simulink library "SimulinkForSyDe"  (R2020b)
settings: Solver=VariableStepAuto  StartTime=0.0  StopTime=10.0  RelTol=1e-3
undefined symbols (not defined in the file): __PRM__SERIALIZED__DATA__, delaynSY
settings Model: Creator=Andrea  LastModifiedBy=Andrea

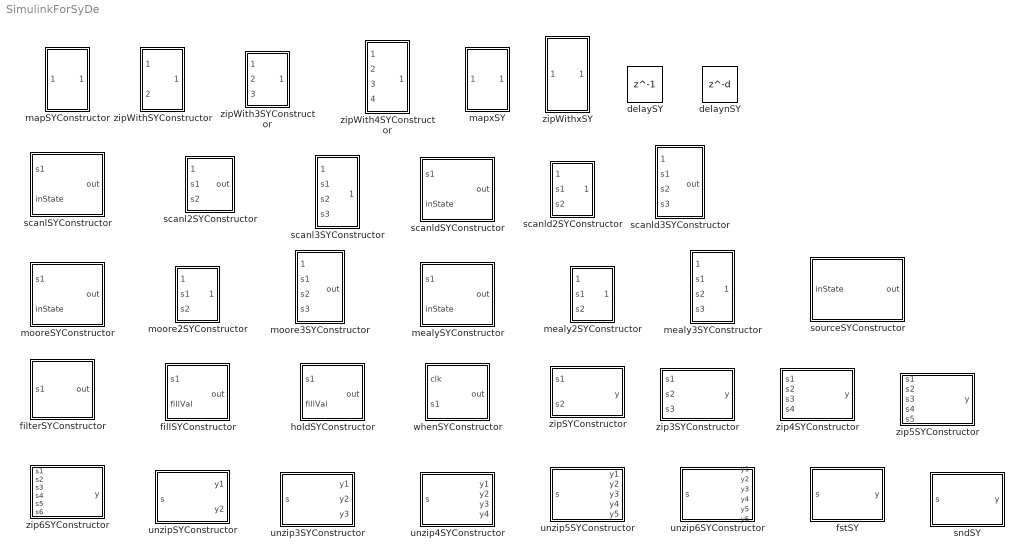
== system SimulinkForSyDe ==
  delaySY : Delay  BlockKeywords=__PRM__SERIALIZED__DATA__:My Integrator  DelayLength=1  InitialConditionSource=Input port
      settings: InputPortMap=u0,p4
  delaynSY : Delay  BlockKeywords=__PRM__SERIALIZED__DATA__:delaynSY  DelayLengthSource=Input port  DelayLength=1  InitialConditionSource=Input port
      settings: InputPortMap=u0,p1,p4
  fillSYConstructor : Stateflow chart  Description="Signals with NaN values cannot be easily imported from Matlab to Simulink and this block need clean signal as input (you  can use cleanNanScript to clean the input signal)."  TreatAsAtomicUnit=on
  filterSYConstructor : Subsystem  Description=The limit must be decided inside the Simulink's function block. The template is equivalent to: filterSY (<=3) s1
  fstSY : MATLAB Function  TreatAsAtomicUnit=on
  holdSYConstructor : Stateflow chart  TreatAsAtomicUnit=on
  mapSYConstructor : Subsystem
  mapxSY : Subsystem  Description=the input must be a mux of signals and the sum is the function used as example
  mealy2SYConstructor : Subsystem
  mealy3SYConstructor : Subsystem
  mealySYConstructor : Subsystem  Description=|
      | The combinational function for next state decoder and for the output have to be set inside this subsystem (disabing the links).
      | This block is a template corresponding to the ForSyDe line of code: mealySY (+) (*) inState $ s1
  moore2SYConstructor : Subsystem
  moore3SYConstructor : Subsystem
  mooreSYConstructor : Subsystem  Description=|
      | The combinational function for next state decoder and for the output have to be set inside this subsystem (disabing the links).
      | This block is a template corresponding to the ForSyDe line of code: mooreSY (+) (*2) inState $ s1.
  scanl2SYConstructor : Subsystem
  scanl3SYConstructor : Subsystem
  scanlSYConstructor : Subsystem  Description=|
      | The combinational function for the output have to be set inside this subsystem (disabing the links).
      | This block is a template corresponding to the ForSyDe line of code: scanlSY (+) inState s1
  scanld2SYConstructor : Subsystem
  scanld3SYConstructor : Subsystem
  scanldSYConstructor : Subsystem  Description=|
      | The combinational function for next state decoder has to be set inside this subsystem (disabing the links).
      | This block is a template corresponding to the ForSyDe line of code: scanldSY (+) inState s1
  sndSY : MATLAB Function  TreatAsAtomicUnit=on
  sourceSYConstructor : Subsystem  Description=The recurrent function has to be changed inside the SImulink's function block. The default template is equivalent to: sourceSY (+1) 0
  unzip3SYConstructor : MATLAB Function  TreatAsAtomicUnit=on
  unzip4SYConstructor : MATLAB Function  TreatAsAtomicUnit=on
  unzip5SYConstructor : MATLAB Function  TreatAsAtomicUnit=on
  unzip6SYConstructor : MATLAB Function  TreatAsAtomicUnit=on
  unzipSYConstructor : MATLAB Function  TreatAsAtomicUnit=on
  whenSYConstructor : Stateflow chart  TreatAsAtomicUnit=on
  zip3SYConstructor : MATLAB Function  TreatAsAtomicUnit=on
  zip4SYConstructor : MATLAB Function  TreatAsAtomicUnit=on
  zip5SYConstructor : MATLAB Function  TreatAsAtomicUnit=on
  zip6SYConstructor : MATLAB Function  TreatAsAtomicUnit=on
  zipSYConstructor : MATLAB Function  TreatAsAtomicUnit=on
  zipWith3SYConstructor : Subsystem
  zipWith4SYConstructor : Subsystem
  zipWithSYConstructor : Subsystem
  zipWithxSY : Subsystem  Description=xSig must be defined before using this block from Matlab and indicates the number of signals contained in the input signals vector

== system SimulinkForSyDe/filterSYConstructor ==
  s1 : Inport
  filterSY : Stateflow chart  TreatAsAtomicUnit=on
  filterf : Subsystem  TreatAsAtomicUnit=on
  out : Outport
  wires:
  filterSY/1(out) -> out/1
  s1/1 -> filterSY/1(s1)

== system SimulinkForSyDe/mapSYConstructor ==
  In1 : Inport
  mapSY : FunctionCaller  FunctionPrototype=y = mapSYf(u)  InputArgumentSpecifications=<Enter example>  OutputArgumentSpecifications=<Enter example>
  mapSY Function : Subsystem  TreatAsAtomicUnit=on
  Out1 : Outport
  wires:
  In1/1 -> mapSY/1
  mapSY/1 -> Out1/1

== system SimulinkForSyDe/mapxSY ==
  In1 : Inport
  Constant : Constant
  Sum : Sum  Inputs=|++
  Out1 : Outport
  wires:
  In1/1 -> Sum/1
  Sum/1 -> Out1/1
  Constant/1 -> Sum/2

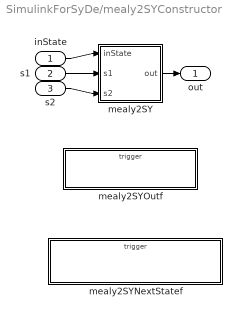
== system SimulinkForSyDe/mealy2SYConstructor ==
  inState : Inport
  s1 : Inport  Port=2
  s2 : Inport  Port=3
  mealy2SY : Stateflow chart  TreatAsAtomicUnit=on
  mealy2SYNextStatef : Subsystem  TreatAsAtomicUnit=on
  mealy2SYOutf : Subsystem  TreatAsAtomicUnit=on
  out : Outport
  wires:
  inState/1 -> mealy2SY/1(inState)
  s1/1 -> mealy2SY/2(s1)
  s2/1 -> mealy2SY/3(s2)
  mealy2SY/1(out) -> out/1

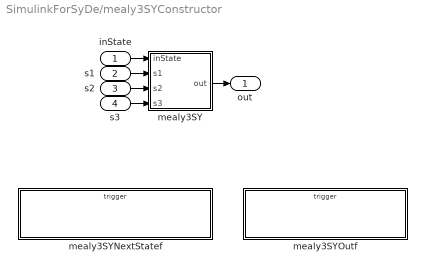
== system SimulinkForSyDe/mealy3SYConstructor ==
  inState : Inport
  s1 : Inport  Port=2
  s2 : Inport  Port=3
  s3 : Inport  Port=4
  mealy3SY : Stateflow chart  TreatAsAtomicUnit=on
  mealy3SYNextStatef : Subsystem  TreatAsAtomicUnit=on
  mealy3SYOutf : Subsystem  TreatAsAtomicUnit=on
  out : Outport
  wires:
  s3/1 -> mealy3SY/4(s3)
  s1/1 -> mealy3SY/2(s1)
  mealy3SY/1(out) -> out/1
  s2/1 -> mealy3SY/3(s2)
  inState/1 -> mealy3SY/1(inState)

== system SimulinkForSyDe/mealySYConstructor ==
  s1 : Inport
  inState : Inport  Port=2
  mealySY : Stateflow chart  TreatAsAtomicUnit=on
  mealySYNextStatef : Subsystem  TreatAsAtomicUnit=on
  mealySYOutf : Subsystem  TreatAsAtomicUnit=on
  out : Outport
  wires:
  mealySY/1(out) -> out/1
  s1/1 -> mealySY/1(s1)
  inState/1 -> mealySY/2(inState)

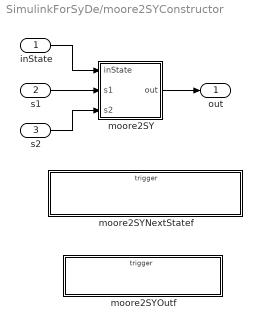
== system SimulinkForSyDe/moore2SYConstructor ==
  inState : Inport
  s1 : Inport  Port=2
  s2 : Inport  Port=3
  moore2SY : Stateflow chart  TreatAsAtomicUnit=on
  moore2SYNextStatef : Subsystem  TreatAsAtomicUnit=on
  moore2SYOutf : Subsystem  TreatAsAtomicUnit=on
  out : Outport
  wires:
  inState/1 -> moore2SY/1(inState)
  s2/1 -> moore2SY/3(s2)
  moore2SY/1(out) -> out/1
  s1/1 -> moore2SY/2(s1)

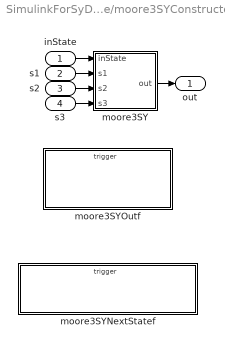
== system SimulinkForSyDe/moore3SYConstructor ==
  inState : Inport
  s1 : Inport  Port=2
  s2 : Inport  Port=3
  s3 : Inport  Port=4
  moore3SY : Stateflow chart  TreatAsAtomicUnit=on
  moore3SYNextStatef : Subsystem  TreatAsAtomicUnit=on
  moore3SYOutf : Subsystem  TreatAsAtomicUnit=on
  out : Outport
  wires:
  moore3SY/1(out) -> out/1
  s1/1 -> moore3SY/2(s1)
  inState/1 -> moore3SY/1(inState)
  s2/1 -> moore3SY/3(s2)
  s3/1 -> moore3SY/4(s3)

== system SimulinkForSyDe/mooreSYConstructor ==
  s1 : Inport
  inState : Inport  Port=2
  mooreSY : Stateflow chart  TreatAsAtomicUnit=on
  mooreSYNextStatef : Subsystem  TreatAsAtomicUnit=on
  mooreSYOutf : Subsystem  TreatAsAtomicUnit=on
  out : Outport
  wires:
  s1/1 -> mooreSY/1(s1)
  inState/1 -> mooreSY/2(inState)
  mooreSY/1(out) -> out/1

== system SimulinkForSyDe/scanl2SYConstructor ==
  inState : Inport
  s1 : Inport  Port=2
  s2 : Inport  Port=3
  scanl2SY : Stateflow chart  TreatAsAtomicUnit=on
  scanl2SYOutf : Subsystem  TreatAsAtomicUnit=on
  out : Outport
  wires:
  s2/1 -> scanl2SY/3(s2)
  inState/1 -> scanl2SY/1(inState)
  s1/1 -> scanl2SY/2(s1)
  scanl2SY/1(out) -> out/1

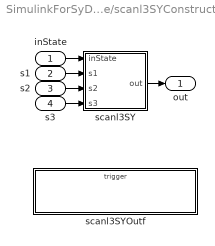
== system SimulinkForSyDe/scanl3SYConstructor ==
  inState : Inport
  s1 : Inport  Port=2
  s2 : Inport  Port=3
  s3 : Inport  Port=4
  scanl3SY : Stateflow chart  TreatAsAtomicUnit=on
  scanl3SYOutf : Subsystem  TreatAsAtomicUnit=on
  out : Outport
  wires:
  s2/1 -> scanl3SY/3(s2)
  s1/1 -> scanl3SY/2(s1)
  inState/1 -> scanl3SY/1(inState)
  scanl3SY/1(out) -> out/1
  s3/1 -> scanl3SY/4(s3)

== system SimulinkForSyDe/scanlSYConstructor ==
  s1 : Inport
  inState : Inport  Port=2
  scanlSY : Stateflow chart  TreatAsAtomicUnit=on
  scanlSYOutf : Subsystem  TreatAsAtomicUnit=on
  out : Outport
  wires:
  scanlSY/1(out) -> out/1
  s1/1 -> scanlSY/1(s1)
  inState/1 -> scanlSY/2(inState)

== system SimulinkForSyDe/scanld2SYConstructor ==
  inState : Inport
  s1 : Inport  Port=2
  s2 : Inport  Port=3
  scanld2SY : Stateflow chart  TreatAsAtomicUnit=on
  scanld2SYNextf : Subsystem  TreatAsAtomicUnit=on
  out : Outport
  wires:
  s1/1 -> scanld2SY/2(s1)
  inState/1 -> scanld2SY/1(inState)
  scanld2SY/1(out) -> out/1
  s2/1 -> scanld2SY/3(s2)

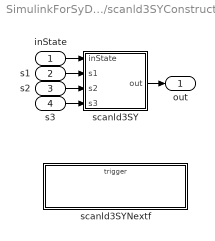
== system SimulinkForSyDe/scanld3SYConstructor ==
  inState : Inport
  s1 : Inport  Port=2
  s2 : Inport  Port=3
  s3 : Inport  Port=4
  scanld3SY : Stateflow chart  TreatAsAtomicUnit=on
  scanld3SYNextf : Subsystem  TreatAsAtomicUnit=on
  out : Outport
  wires:
  s3/1 -> scanld3SY/4(s3)
  s1/1 -> scanld3SY/2(s1)
  s2/1 -> scanld3SY/3(s2)
  scanld3SY/1(out) -> out/1
  inState/1 -> scanld3SY/1(inState)

== system SimulinkForSyDe/scanldSYConstructor ==
  s1 : Inport
  inState : Inport  Port=2
  scanldSY : Stateflow chart  Description=|  TreatAsAtomicUnit=on
      | The combinational function for next state decoder cannot be given as input and the block itself has to be modified to set the wanted decoder function. 
      | This block is a template corresponding to the ForSyDe line of code: scanldSY (+) inState s1
  scanldSYNextf : Subsystem  TreatAsAtomicUnit=on
  out : Outport
  wires:
  s1/1 -> scanldSY/1(s1)
  inState/1 -> scanldSY/2(inState)
  scanldSY/1(out) -> out/1

== system SimulinkForSyDe/sourceSYConstructor ==
  inState : Inport
  To Workspace1 : ToWorkspace  VariableName=yOut  SampleTime=-1
      settings: Save2DSignal=2-D array (concatenate along first dimension)
  recursivef : Subsystem  TreatAsAtomicUnit=on
  sourceSY : Stateflow chart  TreatAsAtomicUnit=on
  out : Outport
  wires:
  inState/1 -> sourceSY/1(inState)
  sourceSY/1(out) -> To Workspace1/1, out/1

== system SimulinkForSyDe/zipWith3SYConstructor ==
  In1 : Inport
  In2 : Inport  Port=2
  In3 : Inport  Port=3
  zipWith3SY : FunctionCaller  FunctionPrototype=y = zipWith3SYf(u,u1,u2)  InputArgumentSpecifications=<Enter example>  OutputArgumentSpecifications=<Enter example>
  zipWith3SY caller : Subsystem  TreatAsAtomicUnit=on
  Out1 : Outport
  wires:
  zipWith3SY/1 -> Out1/1
  In1/1 -> zipWith3SY/1
  In3/1 -> zipWith3SY/3
  In2/1 -> zipWith3SY/2

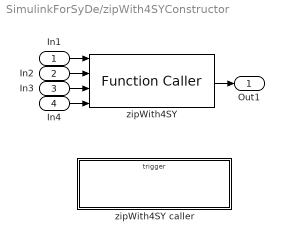
== system SimulinkForSyDe/zipWith4SYConstructor ==
  In1 : Inport
  In2 : Inport  Port=2
  In3 : Inport  Port=3
  In4 : Inport  Port=4
  zipWith4SY : FunctionCaller  FunctionPrototype=y = zipWith4SYf(u,u1,u2,u3)  InputArgumentSpecifications=<Enter example>  OutputArgumentSpecifications=<Enter example>
  zipWith4SY caller : Subsystem  TreatAsAtomicUnit=on
  Out1 : Outport
  wires:
  In2/1 -> zipWith4SY/2
  In1/1 -> zipWith4SY/1
  zipWith4SY/1 -> Out1/1
  In3/1 -> zipWith4SY/3
  In4/1 -> zipWith4SY/4

== system SimulinkForSyDe/zipWithSYConstructor ==
  In1 : Inport
  In2 : Inport  Port=2
  zipWithSY : FunctionCaller  FunctionPrototype=y = zipWithSYf(u,u1)  InputArgumentSpecifications=<Enter example>  OutputArgumentSpecifications=<Enter example>
  zipWithSY caller : Subsystem  TreatAsAtomicUnit=on
  Out1 : Outport
  wires:
  In1/1 -> zipWithSY/1
  zipWithSY/1 -> Out1/1
  In2/1 -> zipWithSY/2

== system SimulinkForSyDe/zipWithxSY ==
  In1 : Inport
  Demux : Demux  Outputs=3
  Sum : Sum  Inputs=+++
  Out3 : Outport
  wires:
  Demux/1 -> Sum/1
  Sum/1 -> Out3/1
  Demux/2 -> Sum/2
  Demux/3 -> Sum/3
  In1/1 -> Demux/1

== system SimulinkForSyDe/filterSYConstructor/filterf ==
  filterf : TriggerPort  TriggerType=function-call  IsSimulinkFunction=on  FunctionName=filterf  FunctionVisibility=scoped  VariantControl=(inherit)
  Constant1 : Constant  Value=3
  Sum : Sum  Inputs=|+-
  u : ArgIn  DisableCoverage=on  ArgumentName=u
  y : ArgOut  DisableCoverage=on  ArgumentName=y
  wires:
  u/1 -> Sum/1
  Constant1/1 -> Sum/2
  Sum/1 -> y/1

== system SimulinkForSyDe/mapSYConstructor/mapSY Function ==
  mapSYf : TriggerPort  TriggerType=function-call  IsSimulinkFunction=on  FunctionName=mapSYf  FunctionVisibility=scoped  VariantControl=(inherit)
  Constant : Constant
  Sum : Sum  Inputs=|++
  u : ArgIn  DisableCoverage=on  ArgumentName=u
  y : ArgOut  DisableCoverage=on  ArgumentName=y
  wires:
  Constant/1 -> Sum/2
  u/1 -> Sum/1
  Sum/1 -> y/1

== system SimulinkForSyDe/mealy2SYConstructor/mealy2SYNextStatef ==
  mealy2SYNextStatef : TriggerPort  TriggerType=function-call  IsSimulinkFunction=on  FunctionName=mealy2SYNextStatef  FunctionVisibility=scoped  VariantControl=(inherit)
  Sum : Sum  Inputs=+++
  u : ArgIn  DisableCoverage=on  ArgumentName=u
  u1 : ArgIn  DisableCoverage=on  Port=2  ArgumentName=u1
  u2 : ArgIn  DisableCoverage=on  Port=3  ArgumentName=u2
  y : ArgOut  DisableCoverage=on  ArgumentName=y
  wires:
  u1/1 -> Sum/2
  Sum/1 -> y/1
  u/1 -> Sum/1
  u2/1 -> Sum/3

== system SimulinkForSyDe/mealy2SYConstructor/mealy2SYOutf ==
  mealy2SYOutf : TriggerPort  TriggerType=function-call  IsSimulinkFunction=on  FunctionName=mealy2SYOutf  FunctionVisibility=scoped  VariantControl=(inherit)
  Sum : Sum  Inputs=+++
  u : ArgIn  DisableCoverage=on  ArgumentName=u
  u1 : ArgIn  DisableCoverage=on  Port=2  ArgumentName=u1
  u2 : ArgIn  DisableCoverage=on  Port=3  ArgumentName=u2
  y : ArgOut  DisableCoverage=on  ArgumentName=y
  wires:
  u1/1 -> Sum/2
  Sum/1 -> y/1
  u/1 -> Sum/1
  u2/1 -> Sum/3

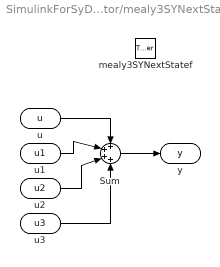
== system SimulinkForSyDe/mealy3SYConstructor/mealy3SYNextStatef ==
  mealy3SYNextStatef : TriggerPort  TriggerType=function-call  IsSimulinkFunction=on  FunctionName=mealy3SYNextStatef  FunctionVisibility=scoped  VariantControl=(inherit)
  Sum : Sum  Inputs=++++
  u : ArgIn  DisableCoverage=on  ArgumentName=u
  u1 : ArgIn  DisableCoverage=on  Port=2  ArgumentName=u1
  u2 : ArgIn  DisableCoverage=on  Port=3  ArgumentName=u2
  u3 : ArgIn  DisableCoverage=on  Port=4  ArgumentName=u3
  y : ArgOut  DisableCoverage=on  ArgumentName=y
  wires:
  u1/1 -> Sum/2
  u/1 -> Sum/1
  u2/1 -> Sum/3
  Sum/1 -> y/1
  u3/1 -> Sum/4

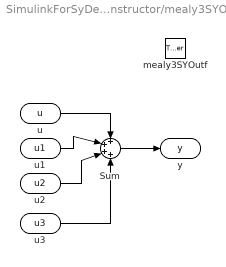
== system SimulinkForSyDe/mealy3SYConstructor/mealy3SYOutf ==
  mealy3SYOutf : TriggerPort  TriggerType=function-call  IsSimulinkFunction=on  FunctionName=mealy3SYOutf  FunctionVisibility=scoped  VariantControl=(inherit)
  Sum : Sum  Inputs=++++
  u : ArgIn  DisableCoverage=on  ArgumentName=u
  u1 : ArgIn  DisableCoverage=on  Port=2  ArgumentName=u1
  u2 : ArgIn  DisableCoverage=on  Port=3  ArgumentName=u2
  u3 : ArgIn  DisableCoverage=on  Port=4  ArgumentName=u3
  y : ArgOut  DisableCoverage=on  ArgumentName=y
  wires:
  u1/1 -> Sum/2
  u/1 -> Sum/1
  u2/1 -> Sum/3
  Sum/1 -> y/1
  u3/1 -> Sum/4

== system SimulinkForSyDe/mealySYConstructor/mealySYNextStatef ==
  mealySYNextStatef : TriggerPort  TriggerType=function-call  IsSimulinkFunction=on  FunctionName=mealySYNextStatef  FunctionVisibility=scoped  VariantControl=(inherit)
  Sum : Sum  Inputs=|++
  u : ArgIn  DisableCoverage=on  ArgumentName=u
  u1 : ArgIn  DisableCoverage=on  Port=2  ArgumentName=u1
  y : ArgOut  DisableCoverage=on  ArgumentName=y
  wires:
  u/1 -> Sum/1
  u1/1 -> Sum/2
  Sum/1 -> y/1

== system SimulinkForSyDe/mealySYConstructor/mealySYOutf ==
  mealySYOutf : TriggerPort  TriggerType=function-call  IsSimulinkFunction=on  FunctionName=mealySYOutf  FunctionVisibility=scoped  VariantControl=(inherit)
  Product : Product
  u : ArgIn  DisableCoverage=on  ArgumentName=u
  u1 : ArgIn  DisableCoverage=on  Port=2  ArgumentName=u1
  y : ArgOut  DisableCoverage=on  ArgumentName=y
  wires:
  u/1 -> Product/1
  u1/1 -> Product/2
  Product/1 -> y/1

== system SimulinkForSyDe/moore2SYConstructor/moore2SYNextStatef ==
  moore2SYNextStatef : TriggerPort  TriggerType=function-call  IsSimulinkFunction=on  FunctionName=moore2SYNextStatef  FunctionVisibility=scoped  VariantControl=(inherit)
  Sum : Sum  Inputs=+++
  u : ArgIn  DisableCoverage=on  ArgumentName=u
  u1 : ArgIn  DisableCoverage=on  Port=2  ArgumentName=u1
  u2 : ArgIn  DisableCoverage=on  Port=3  ArgumentName=u2
  y : ArgOut  DisableCoverage=on  ArgumentName=y
  wires:
  Sum/1 -> y/1
  u1/1 -> Sum/2
  u/1 -> Sum/1
  u2/1 -> Sum/3

== system SimulinkForSyDe/moore2SYConstructor/moore2SYOutf ==
  moore2SYOutf : TriggerPort  TriggerType=function-call  IsSimulinkFunction=on  FunctionName=moore2SYOutf  FunctionVisibility=scoped  VariantControl=(inherit)
  Gain : Gain  Gain=2
  u : ArgIn  DisableCoverage=on  ArgumentName=u
  y : ArgOut  DisableCoverage=on  ArgumentName=y
  wires:
  u/1 -> Gain/1
  Gain/1 -> y/1

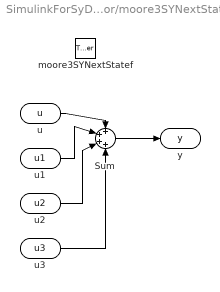
== system SimulinkForSyDe/moore3SYConstructor/moore3SYNextStatef ==
  moore3SYNextStatef : TriggerPort  TriggerType=function-call  IsSimulinkFunction=on  FunctionName=moore3SYNextStatef  FunctionVisibility=scoped  VariantControl=(inherit)
  Sum : Sum  Inputs=++++
  u : ArgIn  DisableCoverage=on  ArgumentName=u
  u1 : ArgIn  DisableCoverage=on  Port=2  ArgumentName=u1
  u2 : ArgIn  DisableCoverage=on  Port=3  ArgumentName=u2
  u3 : ArgIn  DisableCoverage=on  Port=4  ArgumentName=u3
  y : ArgOut  DisableCoverage=on  ArgumentName=y
  wires:
  u1/1 -> Sum/2
  Sum/1 -> y/1
  u2/1 -> Sum/3
  u/1 -> Sum/1
  u3/1 -> Sum/4

== system SimulinkForSyDe/moore3SYConstructor/moore3SYOutf ==
  moore3SYOutf : TriggerPort  TriggerType=function-call  IsSimulinkFunction=on  FunctionName=moore3SYOutf  FunctionVisibility=scoped  VariantControl=(inherit)
  Gain : Gain  Gain=2
  u : ArgIn  DisableCoverage=on  ArgumentName=u
  y : ArgOut  DisableCoverage=on  ArgumentName=y
  wires:
  Gain/1 -> y/1
  u/1 -> Gain/1

== system SimulinkForSyDe/mooreSYConstructor/mooreSYNextStatef ==
  mooreSYNextStatef : TriggerPort  TriggerType=function-call  IsSimulinkFunction=on  FunctionName=mooreSYNextStatef  FunctionVisibility=scoped  VariantControl=(inherit)
  Sum : Sum  Inputs=|++
  u : ArgIn  DisableCoverage=on  ArgumentName=u
  u1 : ArgIn  DisableCoverage=on  Port=2  ArgumentName=u1
  y : ArgOut  DisableCoverage=on  ArgumentName=y
  wires:
  u/1 -> Sum/1
  u1/1 -> Sum/2
  Sum/1 -> y/1

== system SimulinkForSyDe/mooreSYConstructor/mooreSYOutf ==
  mooreSYOutf : TriggerPort  TriggerType=function-call  IsSimulinkFunction=on  FunctionName=mooreSYOutf  FunctionVisibility=scoped  VariantControl=(inherit)
  Gain : Gain  Gain=2
  u : ArgIn  DisableCoverage=on  ArgumentName=u
  y : ArgOut  DisableCoverage=on  ArgumentName=y
  wires:
  u/1 -> Gain/1
  Gain/1 -> y/1

== system SimulinkForSyDe/scanl2SYConstructor/scanl2SYOutf ==
  scanl2SYOutf : TriggerPort  TriggerType=function-call  IsSimulinkFunction=on  FunctionName=scanl2SYOutf  FunctionVisibility=scoped  VariantControl=(inherit)
  Sum : Sum  Inputs=|+++
  u : ArgIn  DisableCoverage=on  ArgumentName=u
  u1 : ArgIn  DisableCoverage=on  Port=2  ArgumentName=u1
  u2 : ArgIn  DisableCoverage=on  Port=3  ArgumentName=u2
  y : ArgOut  DisableCoverage=on  ArgumentName=y
  wires:
  u1/1 -> Sum/2
  u/1 -> Sum/1
  Sum/1 -> y/1
  u2/1 -> Sum/3

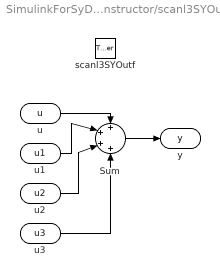
== system SimulinkForSyDe/scanl3SYConstructor/scanl3SYOutf ==
  scanl3SYOutf : TriggerPort  TriggerType=function-call  IsSimulinkFunction=on  FunctionName=scanl3SYOutf  FunctionVisibility=scoped  VariantControl=(inherit)
  Sum : Sum  Inputs=++++
  u : ArgIn  DisableCoverage=on  ArgumentName=u
  u1 : ArgIn  DisableCoverage=on  Port=2  ArgumentName=u1
  u2 : ArgIn  DisableCoverage=on  Port=3  ArgumentName=u2
  u3 : ArgIn  DisableCoverage=on  Port=4  ArgumentName=u3
  y : ArgOut  DisableCoverage=on  ArgumentName=y
  wires:
  u/1 -> Sum/1
  u1/1 -> Sum/2
  Sum/1 -> y/1
  u2/1 -> Sum/3
  u3/1 -> Sum/4

== system SimulinkForSyDe/scanlSYConstructor/scanlSYOutf ==
  scanlSYOutf : TriggerPort  TriggerType=function-call  IsSimulinkFunction=on  FunctionName=scanlSYOutf  FunctionVisibility=scoped  VariantControl=(inherit)
  Sum : Sum  Inputs=|++
  u : ArgIn  DisableCoverage=on  ArgumentName=u
  u1 : ArgIn  DisableCoverage=on  Port=2  ArgumentName=u1
  y : ArgOut  DisableCoverage=on  ArgumentName=y
  wires:
  u/1 -> Sum/1
  u1/1 -> Sum/2
  Sum/1 -> y/1

== system SimulinkForSyDe/scanld2SYConstructor/scanld2SYNextf ==
  scanld2SYNextf : TriggerPort  TriggerType=function-call  IsSimulinkFunction=on  FunctionName=scanld2SYNextf  FunctionVisibility=scoped  VariantControl=(inherit)
  Sum : Sum  Inputs=|+++
  u : ArgIn  DisableCoverage=on  ArgumentName=u
  u1 : ArgIn  DisableCoverage=on  Port=2  ArgumentName=u1
  u2 : ArgIn  DisableCoverage=on  Port=3  ArgumentName=u2
  y : ArgOut  DisableCoverage=on  ArgumentName=y
  wires:
  u/1 -> Sum/1
  Sum/1 -> y/1
  u1/1 -> Sum/2
  u2/1 -> Sum/3

== system SimulinkForSyDe/scanld3SYConstructor/scanld3SYNextf ==
  scanld3SYNextf : TriggerPort  TriggerType=function-call  IsSimulinkFunction=on  FunctionName=scanld3SYNextf  FunctionVisibility=scoped  VariantControl=(inherit)
  Sum : Sum  Inputs=++++
  u : ArgIn  DisableCoverage=on  ArgumentName=u
  u1 : ArgIn  DisableCoverage=on  Port=2  ArgumentName=u1
  u2 : ArgIn  DisableCoverage=on  Port=3  ArgumentName=u2
  u3 : ArgIn  DisableCoverage=on  Port=4  ArgumentName=u3
  y : ArgOut  DisableCoverage=on  ArgumentName=y
  wires:
  Sum/1 -> y/1
  u2/1 -> Sum/3
  u/1 -> Sum/1
  u1/1 -> Sum/2
  u3/1 -> Sum/4

== system SimulinkForSyDe/scanldSYConstructor/scanldSYNextf ==
  scanldSYNextf : TriggerPort  TriggerType=function-call  IsSimulinkFunction=on  FunctionName=scanldSYNextf  FunctionVisibility=scoped  VariantControl=(inherit)
  Sum : Sum  Inputs=|++
  u : ArgIn  DisableCoverage=on  ArgumentName=u
  u1 : ArgIn  DisableCoverage=on  Port=2  ArgumentName=u1
  y : ArgOut  DisableCoverage=on  ArgumentName=y
  wires:
  u/1 -> Sum/1
  u1/1 -> Sum/2
  Sum/1 -> y/1

== system SimulinkForSyDe/sourceSYConstructor/recursivef ==
  recursivef : TriggerPort  TriggerType=function-call  IsSimulinkFunction=on  FunctionName=recursivef  FunctionVisibility=scoped  VariantControl=(inherit)
  Constant : Constant
  Sum : Sum  Inputs=|++
  u : ArgIn  DisableCoverage=on  ArgumentName=u
  y : ArgOut  DisableCoverage=on  ArgumentName=y
  wires:
  Sum/1 -> y/1
  u/1 -> Sum/1
  Constant/1 -> Sum/2

== system SimulinkForSyDe/zipWith3SYConstructor/zipWith3SY caller ==
  zipWith3SYf : TriggerPort  TriggerType=function-call  IsSimulinkFunction=on  FunctionName=zipWith3SYf  FunctionVisibility=scoped  VariantControl=(inherit)
  Sum : Sum  Inputs=|+++
  u : ArgIn  DisableCoverage=on  ArgumentName=u
  u1 : ArgIn  DisableCoverage=on  Port=2  ArgumentName=u1
  u2 : ArgIn  DisableCoverage=on  Port=3  ArgumentName=u2
  y : ArgOut  DisableCoverage=on  ArgumentName=y
  wires:
  u/1 -> Sum/1
  u1/1 -> Sum/2
  u2/1 -> Sum/3
  Sum/1 -> y/1

== system SimulinkForSyDe/zipWith4SYConstructor/zipWith4SY caller ==
  zipWith4SYf : TriggerPort  TriggerType=function-call  IsSimulinkFunction=on  FunctionName=zipWith4SYf  FunctionVisibility=scoped  VariantControl=(inherit)
  Sum : Sum  Inputs=|++++
  u : ArgIn  DisableCoverage=on  ArgumentName=u
  u1 : ArgIn  DisableCoverage=on  Port=2  ArgumentName=u1
  u2 : ArgIn  DisableCoverage=on  Port=3  ArgumentName=u2
  u3 : ArgIn  DisableCoverage=on  Port=4  ArgumentName=u3
  y : ArgOut  DisableCoverage=on  ArgumentName=y
  wires:
  u/1 -> Sum/1
  u1/1 -> Sum/2
  u2/1 -> Sum/3
  u3/1 -> Sum/4
  Sum/1 -> y/1

== system SimulinkForSyDe/zipWithSYConstructor/zipWithSY caller ==
  zipWithSYf : TriggerPort  TriggerType=function-call  IsSimulinkFunction=on  FunctionName=zipWithSYf  FunctionVisibility=scoped  VariantControl=(inherit)
  Sum : Sum  Inputs=|++
  u : ArgIn  DisableCoverage=on  ArgumentName=u
  u1 : ArgIn  DisableCoverage=on  Port=2  ArgumentName=u1
  y : ArgOut  DisableCoverage=on  ArgumentName=y
  wires:
  u1/1 -> Sum/2
  u/1 -> Sum/1
  Sum/1 -> y/1

== stateflow chart SimulinkForSyDe/moore3SYConstructor/moore3SY ==
  state next
    entry:
    locState=inState;
    out=moore3SYOutf(locState);
    locState=moore3SYNextStatef(locState,s1,s2,s3);
    during:
    out=moore3SYOutf(locState);
    locState=moore3SYNextStatef(locState,s1,s2,s3);
  (default) -> next
  data: inState input; s1 input; s2 input; out output; locState local; s3 input

== stateflow chart SimulinkForSyDe/mealy3SYConstructor/mealy3SY ==
  state next
    entry:
    locState=inState;
    out=mealy3SYOutf(locState,s1,s2,s3);
    locState=mealy3SYNextStatef(locState,s1,s2,s3);
    during:
    out=mealy3SYOutf(locState,s1,s2,s3);
    locState=mealy3SYNextStatef(locState,s1,s2,s3);
  (default) -> next
  data: inState input; s1 input; s2 input; s3 input; out output; locState local

== stateflow chart SimulinkForSyDe/sourceSYConstructor/sourceSY ==
  state next
    entry:
    counter=0;
    locState=inState;
    out=locState;
    locState=recursivef(locState);
    counter=counter+1;
    during:
    out=locState;
    locState=recursivef(locState);
    counter=counter+1;
  (default) -> next
  data: inState input; out output; counter local; locState local

== stateflow chart SimulinkForSyDe/filterSYConstructor/filterSY ==
  state Filter
    entry:
    out=filterf(s1)
    if out <= 0
    out = NaN;
    else
    out=s1;
    end
    during:
    out=filterf(s1)
    if out <= 0
    out = NaN;
    else
    out=s1;
    end
  (default) -> Filter
  data: s1 input; out output

== stateflow chart SimulinkForSyDe/scanldSYConstructor/scanldSY ==
  state next
    entry:
    locState=inState;
    out=locState;
    locState=scanldSYNextf(out,s1);
    during:
    out=locState;
    locState=scanldSYNextf(out,s1);
  (default) -> next
  data: out output; locState local; s1 input; inState input

== stateflow chart SimulinkForSyDe/fillSYConstructor ==
  state fill
    if s1==-1
    out=fillVal;
    else
    out=s1;
    end
  (default) -> fill
  data: out output; s1 input; fillVal input

== stateflow chart SimulinkForSyDe/holdSYConstructor ==
  state hold
    entry:
    localVal=fillVal;
    if s1==-1
    out=localVal;
    else
    out=s1;
    localVal=s1;
    end
    during:
    if s1==-1
    out=localVal;
    else
    out=s1;
    localVal=s1;
    end
  (default) -> hold
  data: s1 input; fillVal input; out output; localVal local

== stateflow chart SimulinkForSyDe/whenSYConstructor ==
  state testwhenSY
    if clk==-1
    out=NaN;
    else
    out=s1;
    end
  (default) -> testwhenSY
  data: clk input; out output; s1 input

== matlab function SimulinkForSyDe/zipSYConstructor ==
  data: s1 input; y output; s2 input
function y = fcn(s1,s2)
counterMat=1;
A = zeros(counterMat,2);
A(counterMat,1) = s1;
A(counterMat,2) = s2;
counterMat=counterMat+1;
y=A;

== matlab function SimulinkForSyDe/zip3SYConstructor ==
  data: s1 input; y output; s2 input; s3 input
function y = fcn(s1,s2,s3)
counterMat=1;
A = zeros(counterMat,3);
A(counterMat,1) = s1;
A(counterMat,2) = s2;
A(counterMat,3) = s3;
counterMat=counterMat+1;
y=A;

== matlab function SimulinkForSyDe/zip4SYConstructor ==
  data: s1 input; y output; s2 input; s3 input; s4 input
function y = fcn(s1,s2,s3,s4)
counterMat=1;
A = zeros(counterMat,4);
A(counterMat,1) = s1;
A(counterMat,2) = s2;
A(counterMat,3) = s3;
A(counterMat,4) = s4;
counterMat=counterMat+1;
y=A;

== matlab function SimulinkForSyDe/zip5SYConstructor ==
  data: s1 input; y output; s2 input; s3 input; s4 input; s5 input
function y = fcn(s1,s2,s3,s4,s5)
counterMat=1;
A = zeros(counterMat,5);
A(counterMat,1) = s1;
A(counterMat,2) = s2;
A(counterMat,3) = s3;
A(counterMat,4) = s4;
A(counterMat,5) = s5;
counterMat=counterMat+1;
y=A;

== matlab function SimulinkForSyDe/zip6SYConstructor ==
  data: s1 input; y output; s2 input; s3 input; s4 input; s5 input; s6 input
function y = fcn(s1,s2,s3,s4,s5,s6)
counterMat=1;
A = zeros(counterMat,6);
A(counterMat,1) = s1;
A(counterMat,2) = s2;
A(counterMat,3) = s3;
A(counterMat,4) = s4;
A(counterMat,5) = s5;
A(counterMat,6) = s6;
counterMat=counterMat+1;
y=A;

== matlab function SimulinkForSyDe/unzipSYConstructor ==
  data: s input; y1 output; y2 output
function [y1,y2] = fcn(s)
counterMat=1;
y1=s(counterMat,1);
y2=s(counterMat,2);
counterMat=counterMat+1;

== stateflow chart SimulinkForSyDe/mooreSYConstructor/mooreSY ==
  state next
    entry:
    locState=inState;
    out=mooreSYOutf(locState);
    locState=mooreSYNextStatef(locState,s1);
    during:
    out=mooreSYOutf(locState);
    locState=mooreSYNextStatef(locState,s1);
  (default) -> next
  data: out output; locState local; s1 input; inState input

== matlab function SimulinkForSyDe/unzip3SYConstructor ==
  data: s input; y1 output; y2 output; y3 output
function [y1,y2,y3] = fcn(s)
counterMat=1;
y1=s(counterMat,1);
y2=s(counterMat,2);
y3=s(counterMat,3);
counterMat=counterMat+1;

== matlab function SimulinkForSyDe/unzip4SYConstructor ==
  data: s input; y1 output; y2 output; y3 output; y4 output
function [y1,y2,y3,y4] = fcn(s)
counterMat=1;
y1=s(counterMat,1);
y2=s(counterMat,2);
y3=s(counterMat,3);
y4=s(counterMat,4);
counterMat=counterMat+1;

== matlab function SimulinkForSyDe/unzip5SYConstructor ==
  data: s input; y1 output; y2 output; y3 output; y4 output; y5 output
function [y1,y2,y3,y4,y5] = fcn(s)
counterMat=1;
y1=s(counterMat,1);
y2=s(counterMat,2);
y3=s(counterMat,3);
y4=s(counterMat,4);
y5=s(counterMat,5);
counterMat=counterMat+1;

== matlab function SimulinkForSyDe/unzip6SYConstructor ==
  data: s input; y1 output; y2 output; y3 output; y4 output; y5 output; y6 output
function [y1,y2,y3,y4,y5,y6] = fcn(s)
counterMat=1;
y1=s(counterMat,1);
y2=s(counterMat,2);
y3=s(counterMat,3);
y4=s(counterMat,4);
y5=s(counterMat,5);
y6=s(counterMat,6);
counterMat=counterMat+1;

== matlab function SimulinkForSyDe/fstSY ==
  data: s input; y output
function y= fcn(s)
counterMat=1;
y=s(counterMat,1);
counterMat=counterMat+1;

== matlab function SimulinkForSyDe/sndSY ==
  data: s input; y output
function y= fcn(s)
counterMat=1;
y=s(counterMat,2);
counterMat=counterMat+1;

== stateflow chart SimulinkForSyDe/scanlSYConstructor/scanlSY ==
  state next
    entry:
    locState=inState;
    out=scanlSYOutf(locState,s1);
    locState=out;
    during:
    out=scanlSYOutf(locState,s1);
    locState=out;
  (default) -> next
  data: out output; locState local; s1 input; inState input

== stateflow chart SimulinkForSyDe/mealySYConstructor/mealySY ==
  state next
    entry:
    locState=inState;
    out=mealySYOutf(locState,s1);
    locState=mealySYNextStatef(locState,s1);
    during:
    out=mealySYOutf(locState,s1);
    locState=mealySYNextStatef(locState,s1);
  (default) -> next
  data: s1 input; out output; locState local; inState input

== stateflow chart SimulinkForSyDe/scanl3SYConstructor/scanl3SY ==
  state next
    entry:
    locState=inState;
    out=scanl3SYOutf(locState,s1,s2,s3);
    locState=out;
    during:
    out=scanl3SYOutf(locState,s1,s2,s3);
    locState=out;
  (default) -> next
  data: inState input; s1 input; s2 input; s3 input; locState local; out output

== stateflow chart SimulinkForSyDe/scanl2SYConstructor/scanl2SY ==
  state next
    entry:
    locState=inState;
    out=scanl2SYOutf(locState,s1,s2);
    locState=out;
    during:
    out=scanl2SYOutf(locState,s1,s2);
    locState=out;
  (default) -> next
  data: inState input; s1 input; s2 input; out output; locState local

== stateflow chart SimulinkForSyDe/scanld2SYConstructor/scanld2SY ==
  state next
    entry:
    locState=inState;
    out=locState;
    locState=scanld2SYNextf(out,s1,s2);
    during:
    out=locState;
    locState=scanld2SYNextf(out,s1,s2);
  (default) -> next
  data: inState input; s1 input; s2 input; locState local; out output

== stateflow chart SimulinkForSyDe/scanld3SYConstructor/scanld3SY ==
  state next
    entry:
    locState=inState;
    out=locState;
    locState=scanld3SYNextf(out,s1,s2,s3);
    during:
    out=locState;
    locState=scanld3SYNextf(out,s1,s2,s3);
  (default) -> next
  data: inState input; s1 input; s2 input; s3 input; locState local; out output

== stateflow chart SimulinkForSyDe/moore2SYConstructor/moore2SY ==
  state next
    entry:
    locState=inState;
    out=moore2SYOutf(locState);
    locState=moore2SYNextStatef(locState,s1,s2);
    during:
    out=moore2SYOutf(locState);
    locState=moore2SYNextStatef(locState,s1,s2);
  (default) -> next
  data: inState input; s1 input; s2 input; out output; locState local

== stateflow chart SimulinkForSyDe/mealy2SYConstructor/mealy2SY ==
  state next
    entry:
    locState=inState;
    out=mealy2SYOutf(locState,s1,s2);
    locState=mealy2SYNextStatef(locState,s1,s2);
    during:
    out=mealy2SYOutf(locState,s1,s2);
    locState=mealy2SYNextStatef(locState,s1,s2);
  (default) -> next
  data: inState input; locState local; out output; s1 input; s2 input
